simulink model "Collision_08_Compare_Forces"  (R2014a)
settings: Solver=ode15s  StartTime=0.0  StopTime=5  MaxStep=1e-3  RelTol=1e-8  AbsTol=1e-8
PostLoadFcn:
  | warning off Simulink:Engine:UsingDefaultMaxStepSize
StartFcn:
  | tic;
StopFcn:
  | Elapsed_Sim_Time = toc;
  | disp(['Elapsed Sim Time = ' num2str(Elapsed_Sim_Time)]);
undefined symbols (not defined in the file): Extr_Data_Ring, X, Y, Z
libraries: sm_lib x39, nesl_utility x6, Contact_Forces_Lib x5
(part 2 of 2)

== system Collision_08_Compare_Forces/Subsystem1 ==
  In1 : Inport
  Bus Selector : BusSelector  OutputSignals=Normal Force
  Contact Force : Scope
      settings: YMin=0  YMax=2000  SaveName=ScopeData3
  wires:
  In1/1 -> Bus Selector/1
  Bus Selector/1 -> Contact Force/1  "<Normal Force>"

== system Collision_08_Compare_Forces/Subsystem2 ==
  In1 : Inport
  Bus Selector : BusSelector  OutputSignals=Normal Force
  Contact Force : Scope
      settings: YMin=0  YMax=2000  SaveName=ScopeData3
  wires:
  In1/1 -> Bus Selector/1
  Bus Selector/1 -> Contact Force/1  "<Normal Force>"

== system Collision_08_Compare_Forces/Subsystem3 ==
  In1 : Inport
  Bus Selector : BusSelector  OutputSignals=Normal Force  OutputAsBus=on
  Contact Force : Scope
      settings: YMin=0  YMax=2000
  wires:
  In1/1 -> Bus Selector/1
  Bus Selector/1 -> Contact Force/1

== system Collision_08_Compare_Forces/Subsystem4 ==
  In1 : Inport
  Bus Selector : BusSelector  OutputSignals=Normal Force
  Contact Force : Scope
      settings: YMin=0  YMax=2000  SaveName=ScopeData3
  wires:
  In1/1 -> Bus Selector/1
  Bus Selector/1 -> Contact Force/1  "<Normal Force>"
